simulink model "Trial_Merge_Unsuccessful"  (R2020b)
settings: Solver=VariableStepAuto  StartTime=0.0  StopTime=10.0  RelTol=1e-3
values from neighbouring files (symbols this model uses):
  A_2 = zeros(3)    [MPC_tune.m]
  B_2 = I_inv    [MPC_tune.m]
  C_2 = eye(3)    [MPC_tune.m]
  D_2 = zeros(3)    [MPC_tune.m]
  I_inv = inv(I_mat)    [MPC_tune.m]
undefined symbols (not defined in the file or in its folder): Fb1_l, Fb1_u, Fb2_l, Fb2_u, Fb3_l, Fb3_u, Fb4_l, Fb4_u, Fc1_l, Fc1_u, Fc2_l, Fc2_u, Fc3_l, Fc3_u, fprop, Ft1_l, Ft1_u, Ft2_l, Ft2_u, Ft3_l, Ft3_u, Ft4_l, Ft4_u, theta0
libraries: dspsigops x33, pid_lib x3, fuzblock x3, mpclib x1, dspmathops x1
(part 1 of 2)
settings Model: Creator=Jonathan van Zyl  LastModifiedBy=Jonathan van Zyl

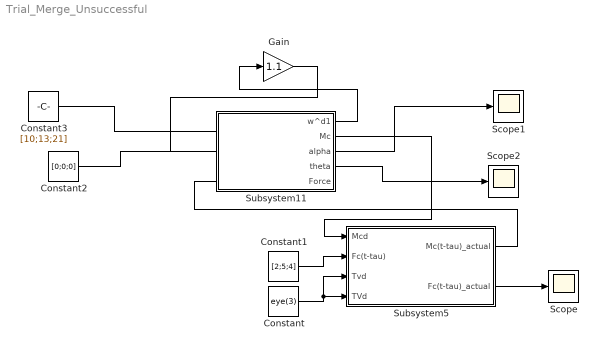
== system Trial_Merge_Unsuccessful ==
  Constant : Constant  Value=eye(3)
  Constant1 : Constant  Value=[2;5;4]
  Constant2 : Constant  Value=[0;0;0]
  Constant3 : Constant  Value=[10;13;21]
  Gain : Gain  Gain=1.1
  Scope : Scope
  Scope1 : Scope
  Scope2 : Scope
  Subsystem11 : Subsystem
  Subsystem5 : Subsystem
  wires:
  Subsystem11/2(Mc) -> Subsystem5/1(Mcd)
  Subsystem5/2(Fc(t-tau)_actual) -> Scope/1
  Constant/1 -> Subsystem5/4(TVd), Subsystem5/3(Tvd)
  Constant1/1 -> Subsystem5/2(Fc(t-tau))
  Subsystem11/1(w^d1) -> Gain/1
  Gain/1 -> ?
  Subsystem5/1(Mc(t-tau)_actual) -> ?
  Constant2/1 -> ?
  Constant3/1 -> ?
  Subsystem11/3(alpha) -> Scope1/1
  Subsystem11/4(theta) -> Scope2/1

== system Trial_Merge_Unsuccessful/Subsystem11 ==
  Add : Sum  Inputs=+++
  Constant : Constant  Value=[0;0;0]
  Constant1 : Constant  Value=[2;3;4]
  Demux : Demux  Outputs=3
  Gain3 : Gain  Gain=180/pi
  M_aero : Constant  Value=[2;3;4]
  Scope : Scope
  Scope1 : Scope
  Scope8 : Scope
  Square : Math  Operator=square  SaturateOnIntegerOverflow=on
  Square Root : Sqrt  SaturateOnIntegerOverflow=on
  Square1 : Math  Operator=square  SaturateOnIntegerOverflow=on
  Square2 : Math  Operator=square  SaturateOnIntegerOverflow=on
  Subsystem : Subsystem
  To Workspace : ToWorkspace  VariableName=angle_deg  SaveFormat=Timeseries  SampleTime=-1
  To Workspace1 : ToWorkspace  VariableName=alpha  SaveFormat=Timeseries  SampleTime=-1
  initial w : Constant  Value=[0;0;0]
  sigma,upsilon,tau : Constant  Value=[2;3;4]
  w^d1 : Outport
  Mc : Outport  Port=2
  alpha : Outport  Port=3
  theta : Outport  Port=4
  Force : Outport  Port=5
  wires:
  Subsystem/4(alpha) -> Demux/1, Scope/1, alpha/1
  Demux/1 -> Square/1
  Demux/2 -> Square1/1
  Demux/3 -> Square2/1
  Square/1 -> Add/1
  Square1/1 -> Add/2
  Square2/1 -> Add/3
  Add/1 -> Square Root/1
  Square Root/1 -> To Workspace1/1, Scope1/1
  sigma,upsilon,tau/1 -> Subsystem/2(sigma,tau,upsilon)
  initial w/1 -> Subsystem/3(initial w)
  M_aero/1 -> Subsystem/1(M_aero)
  Subsystem/3(Mc) -> Mc/1
  Subsystem/2(w_out) -> w^d1/1
  Subsystem/1(theta_out) -> Gain3/1, theta/1
  Gain3/1 -> To Workspace/1, Scope8/1
  Subsystem/5(Force) -> Force/1
  Constant/1 -> Subsystem/4(Fc)
  Constant1/1 -> Subsystem/5(a)

== system Trial_Merge_Unsuccessful/Subsystem5 ==
  Mcd : Inport
  Fc(t-tau) : Inport  Port=2
  Tvd : Inport  Port=3
  TVd : Inport  Port=4
  Gain6 : Gain
  MATLAB Function4 : MATLAB Function  Commented=on  TreatAsAtomicUnit=on
  MATLAB Function5 : MATLAB Function  Commented=on  TreatAsAtomicUnit=on
  Matrix Multiply5 : Product  Multiplication=Matrix(*)
  Scope16 : Scope
  Scope17 : Scope
  Scope18 : Scope
  Subsystem : Subsystem
  Subsystem1 : Subsystem
  Subsystem2 : Subsystem
  Subsystem3 : Subsystem
  Subsystem4 : Subsystem
  Turn off for PID tune : Gain
  Mc(t-tau)_actual : Outport
  Fc(t-tau)_actual : Outport  Port=2
  wires:
  Mcd/1 -> Gain6/1
  Turn off for PID tune/1 -> Matrix Multiply5/2
  Tvd/1 -> Matrix Multiply5/1
  Fc(t-tau)/1 -> Turn off for PID tune/1
  MATLAB Function5/1(F1) -> MATLAB Function4/1(F1)
  MATLAB Function5/3(F3) -> MATLAB Function4/3(F3)
  MATLAB Function5/2(F2) -> MATLAB Function4/2(F2)
  Matrix Multiply5/1 -> Subsystem/1(F_c_d)  "F_c_d"
  Gain6/1 -> Subsystem/2(M_c_d)  "M_c_d"
  Subsystem/1(Fb_wanted) -> Subsystem1/1(In1)
  Subsystem/2(Ft_wanted) -> Subsystem1/2(In2)
  Subsystem/3(Fc_wanted) -> Subsystem1/3(In3)
  Subsystem1/1(Out1) -> Subsystem2/1(In1)
  Subsystem1/2(Out2) -> Subsystem2/2(In2)
  Subsystem1/3(Out3) -> Subsystem2/3(In3)
  Subsystem3/1(Out1) -> Scope17/1, Subsystem4/2(In2)
  Subsystem2/1(F_c_max) -> Subsystem3/1(In1)
  Subsystem2/2(F_t_max) -> Subsystem3/2(In2)
  Subsystem2/3(Out3) -> Subsystem3/3(In3)
  Subsystem2/4(Out4) -> Subsystem3/4(Ft3)
  Subsystem2/5(Out5) -> Subsystem3/5(Ft4)
  Subsystem2/6(Out6) -> Subsystem3/6(Fb1)
  Subsystem2/7(Out7) -> Subsystem3/7(In7)
  Subsystem2/8(Out8) -> Subsystem3/8(Fb3)
  Subsystem2/9(Out9) -> Subsystem3/9(In9)
  Subsystem3/2(Mc(t-tau)_actual) -> Mc(t-tau)_actual/1
  Subsystem4/1(Fc(t-tau)_actual) -> Scope16/1, Fc(t-tau)_actual/1
  TVd/1 -> Subsystem4/1(TVd)
  Subsystem4/2(Fc(t-tau)_actual1) -> Scope18/1

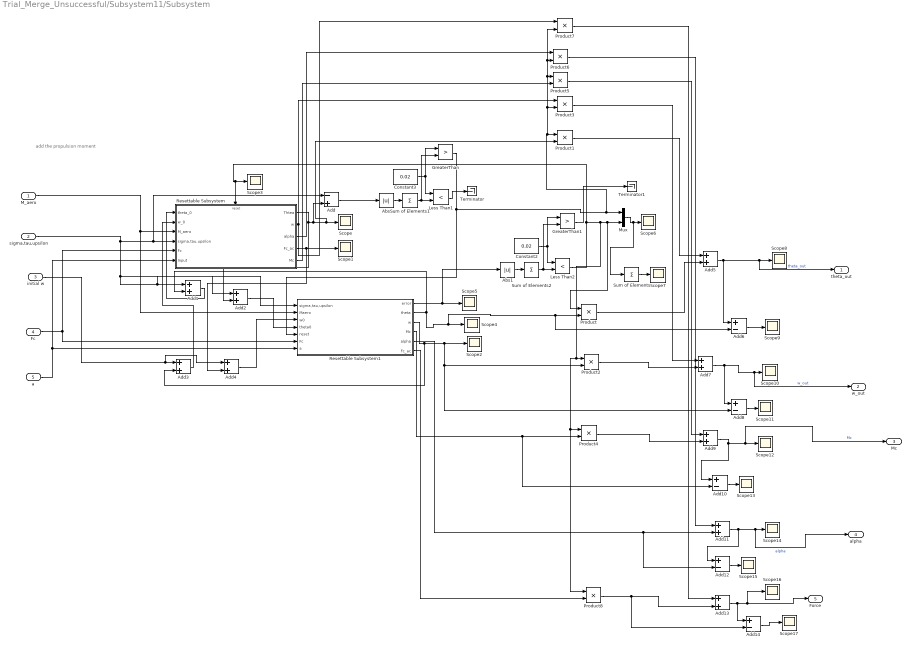
== system Trial_Merge_Unsuccessful/Subsystem11/Subsystem ==
  note: add the propulsion moment
  M_aero : Inport
  sigma,tau,upsilon : Inport  Port=2
  initial w : Inport  Port=3
  Fc : Inport  Port=4
  a : Inport  Port=5
  Abs : Abs
  Abs1 : Abs
  Add : Sum  Inputs=-+
  Add{1..5,7,9,11,13} (9 alike) : Sum
  Add{6,8,10,12,14} (5 alike) : Sum  Inputs=+-
  Constant2 : Constant  Value=0.02
  Constant3 : Constant  Value=0.02
  GreaterThan : RelationalOperator  Operator=>  OutDataTypeStr=boolean  RndMeth=Simplest
  GreaterThan1 : RelationalOperator  Operator=>  OutDataTypeStr=boolean  RndMeth=Simplest
  Less Than1 : RelationalOperator  Operator=<  OutDataTypeStr=boolean  RndMeth=Simplest
  Less Than2 : RelationalOperator  Operator=<  OutDataTypeStr=boolean  RndMeth=Simplest
  Mux : Mux  Inputs=2
  Product{,1..8} (9 alike) : Product
  Resettable Subsystem : Subsystem  TreatAsAtomicUnit=on
  Resettable Subsystem1 : Subsystem  TreatAsAtomicUnit=on
  Scope{,1..17} (18 alike) : Scope
  Sum of Elements : Sum  Inputs=+
  Sum of Elements1 : Sum  Inputs=+
  Sum of Elements2 : Sum  Inputs=+
  Terminator : Terminator
  Terminator1 : Terminator
  theta_out : Outport
  w_out : Outport  Port=2
  Mc : Outport  Port=3
  alpha : Outport  Port=4
  Force : Outport  Port=5
  wires:
  Add8/1 -> Scope11/1
  GreaterThan/1 -> Product7/2, Product6/2, Product5/1, Product3/2, Product1/1, Mux/1, Resettable Subsystem1/5(reset)
  Add6/1 -> Scope9/1
  Abs1/1 -> Sum of Elements2/1
  Product1/1 -> Add5/1
  Resettable Subsystem/2(w) -> Scope1/1, Add4/2, Product3/1
  Resettable Subsystem1/4(Mc) -> Add10/2, Product4/2
  Resettable Subsystem1/2(theta) -> Add1/2, Add6/2, Product/2, Scope4/1
  Resettable Subsystem1/5(alpha) -> Add12/2, Add11/2
  Resettable Subsystem/1(Thtea) -> Add2/2, Add/2, Product1/2, Scope/1
  Less Than2/1 -> Product2/1, Product8/1, Product4/1, Product/1, Mux/2, Scope3/1, Resettable Subsystem/Reset
  M_aero/1 -> Resettable Subsystem1/2(Maero), Resettable Subsystem/3(M_aero)
  Resettable Subsystem1/1(error) -> Abs1/1, Scope5/1
  Add11/1 -> Add12/1, alpha/1, Scope14/1  "alpha"
  Product2/1 -> Add7/2
  Constant2/1 -> GreaterThan1/1, Less Than2/1
  Resettable Subsystem1/3(w) -> Add3/2, Scope2/1, Add8/2, Product2/2
  Product3/1 -> Add7/1
  Add12/1 -> Scope15/1
  Abs/1 -> Sum of Elements1/1
  Add5/1 -> Add6/1, theta_out/1, Scope8/1  "theta_out"
  Add2/1 -> Resettable Subsystem1/4(theta0)
  Constant3/1 -> GreaterThan/1, Less Than1/1
  Sum of Elements1/1 -> Less Than1/2, GreaterThan/2
  Add3/1 -> Resettable Subsystem/2(w_0)
  sigma,tau,upsilon/1 -> Add2/1, Add1/1, Resettable Subsystem1/1(sigma,tau,upsilon), Add/1, Resettable Subsystem/4(sigma,tau,upsilon)
  Product5/1 -> Add9/1
  Resettable Subsystem/5(Mc) -> Product5/2
  Add7/1 -> Add8/1, w_out/1, Scope10/1  "w_out"
  Product6/1 -> Add11/1
  Add9/1 -> Add10/1, Mc/1, Scope12/1  "Mc"
  Add/1 -> Abs/1
  Add1/1 -> Resettable Subsystem/1(theta_0)
  Sum of Elements/1 -> Scope7/1
  Sum of Elements2/1 -> Less Than2/2, GreaterThan1/2
  Mux/1 -> Sum of Elements/1, Scope6/1
  Resettable Subsystem/3(alpha) -> Product6/1
  Add4/1 -> Resettable Subsystem1/3(w0)
  initial w/1 -> Add4/1, Add3/1
  Product/1 -> Add5/2
  Add10/1 -> Scope13/1
  Product4/1 -> Add9/2
  GreaterThan1/1 -> Terminator1/1
  Less Than1/1 -> Terminator/1
  Resettable Subsystem/4(Fc_ac) -> Product7/1
  Fc/1 -> Resettable Subsystem/5(Fc), Resettable Subsystem1/6(Fc)
  a/1 -> Resettable Subsystem1/7(a), Resettable Subsystem/6(Input)
  Resettable Subsystem1/6(Fc_ac) -> Product8/2
  Product8/1 -> Add14/2, Add13/2
  Product7/1 -> Add13/1
  Add13/1 -> Add14/1, Force/1, Scope16/1
  Add14/1 -> Scope17/1

== system Trial_Merge_Unsuccessful/Subsystem5/Subsystem ==
  F_c_d : Inport
  M_c_d : Inport  Port=2
  Demux8 : Demux  Outputs=3
  Demux9 : Demux  Outputs=3
  MATLAB Function : MATLAB Function  TreatAsAtomicUnit=on
  MATLAB Function6 : MATLAB Function  TreatAsAtomicUnit=on
  Mux23 : Mux
  Mux24 : Mux
  Mux9 : Mux  Inputs=3
  Terminator12 : Terminator
  To Workspace6 : ToWorkspace  VariableName=Fc_wanted  SaveFormat=Timeseries  SampleTime=-1
  To Workspace7 : ToWorkspace  VariableName=Ft_wanted  SaveFormat=Timeseries  SampleTime=-1
  To Workspace8 : ToWorkspace  VariableName=Fb_wanted  SaveFormat=Timeseries  SampleTime=-1
  Fb_wanted : Outport
  Ft_wanted : Outport  Port=2
  Fc_wanted : Outport  Port=3
  wires:
  Demux9/3 -> MATLAB Function6/3(M_z)
  Demux8/2 -> MATLAB Function6/1(F_y)
  Mux9/1 -> Fc_wanted/1, To Workspace6/1  "Fc_wanted"
  MATLAB Function/2(Ft2) -> Mux23/2  "Fb_wanted"
  Demux9/1 -> MATLAB Function6/2(M_x)
  MATLAB Function/3(Ft3) -> Mux23/3
  Demux9/2 -> MATLAB Function/1(My)
  MATLAB Function/8(Fb4) -> Mux24/4
  MATLAB Function6/1(F_c1) -> Mux9/1
  MATLAB Function/1(Ft1) -> Mux23/1  "Ft_wanted"
  Demux8/1 -> Terminator12/1
  Mux23/1 -> Ft_wanted/1, To Workspace7/1  "Ft_wanted"
  Mux24/1 -> Fb_wanted/1, To Workspace8/1  "Fb_wanted"
  MATLAB Function6/3(F_c3) -> Mux9/3
  MATLAB Function/5(Fb1) -> Mux24/1
  MATLAB Function/6(Fb2) -> Mux24/2
  MATLAB Function/7(Fb3) -> Mux24/3
  MATLAB Function/4(Ft4) -> Mux23/4
  Demux8/3 -> MATLAB Function/2(Fz)
  MATLAB Function6/2(F_c2) -> Mux9/2
  F_c_d/1 -> Demux8/1
  M_c_d/1 -> Demux9/1

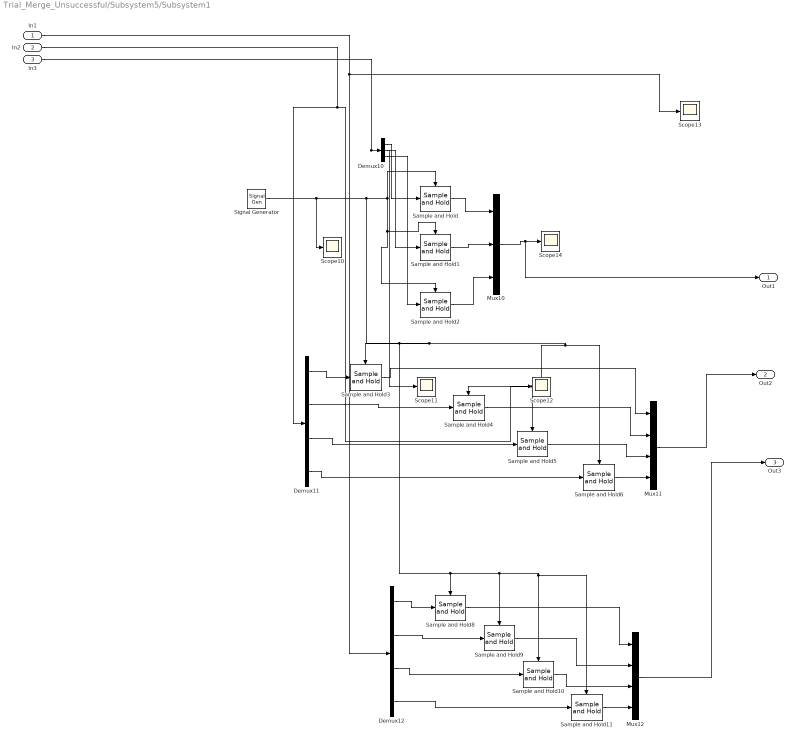
== system Trial_Merge_Unsuccessful/Subsystem5/Subsystem1 ==
  In1 : Inport
  In2 : Inport  Port=2
  In3 : Inport  Port=3
  Demux10 : Demux  Outputs=3
  Demux11 : Demux
  Demux12 : Demux
  Mux10 : Mux  Inputs=3
  Mux11 : Mux
  Mux12 : Mux
  Sample and Hold{,1..6,8..11} (11 alike) : dspsigops/Sample and Hold  trig=Rising edge  initCond=0  latchinput=off
  Scope{10..14} (5 alike) : Scope
  Signal Generator : SignalGenerator  WaveForm=square  Frequency=fprop  Units=rad/sec
  Out1 : Outport
  Out2 : Outport  Port=2
  Out3 : Outport  Port=3
  wires:
  Demux12/1 -> Sample and Hold8/1
  Demux11/1 -> Sample and Hold3/1
  Signal Generator/1 -> Scope10/1, Sample and Hold11/Trigger, Sample and Hold10/Trigger, Sample and Hold9/Trigger, Sample and Hold8/Trigger, Sample and Hold4/Trigger, Sample and Hold5/Trigger, Sample and Hold6/Trigger, Sample and Hold3/Trigger, Sample and Hold/Trigger, Sample and Hold2/Trigger, Sample and Hold1/Trigger
  In2/1 -> Scope12/1, Demux11/1
  In3/1 -> Scope11/1, Demux10/1
  Demux10/3 -> Sample and Hold2/1
  Sample and Hold10/1 -> Mux12/3
  Sample and Hold/1 -> Mux10/1
  Demux12/4 -> Sample and Hold11/1
  Sample and Hold6/1 -> Mux11/4
  Demux10/1 -> Sample and Hold/1
  Mux10/1 -> Out1/1, Scope14/1
  Demux12/3 -> Sample and Hold10/1
  Sample and Hold8/1 -> Mux12/1
  Sample and Hold3/1 -> Mux11/1
  Sample and Hold5/1 -> Mux11/3
  Sample and Hold1/1 -> Mux10/2
  Sample and Hold11/1 -> Mux12/4
  In1/1 -> Scope13/1, Demux12/1
  Demux10/2 -> Sample and Hold1/1
  Demux11/2 -> Sample and Hold4/1
  Sample and Hold2/1 -> Mux10/3
  Sample and Hold4/1 -> Mux11/2
  Sample and Hold9/1 -> Mux12/2
  Demux11/3 -> Sample and Hold5/1
  Mux12/1 -> Out3/1
  Demux12/2 -> Sample and Hold9/1
  Demux11/4 -> Sample and Hold6/1
  Mux11/1 -> Out2/1

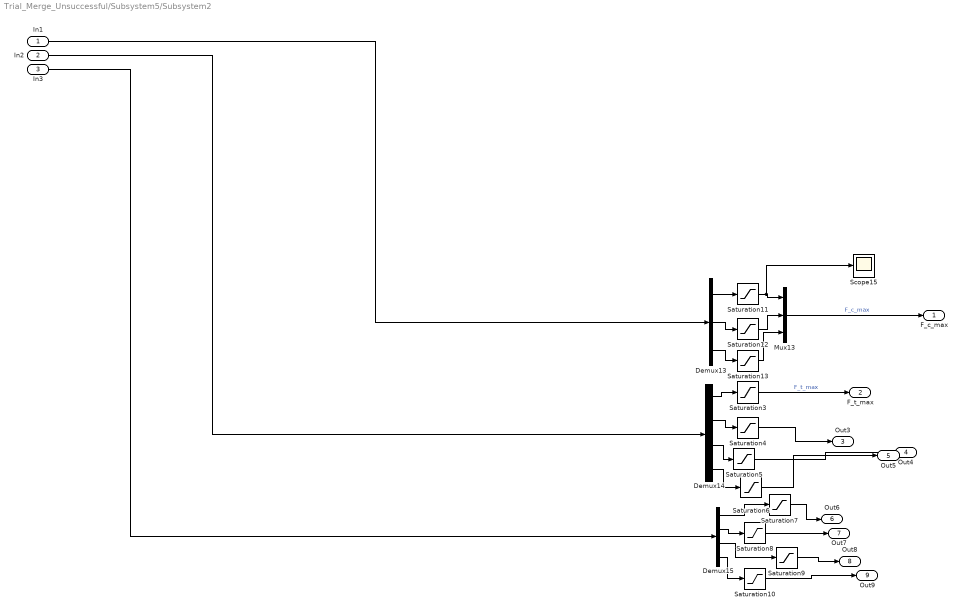
== system Trial_Merge_Unsuccessful/Subsystem5/Subsystem2 ==
  In1 : Inport
  In2 : Inport  Port=2
  In3 : Inport  Port=3
  Demux13 : Demux  Outputs=3
  Demux14 : Demux
  Demux15 : Demux
  Mux13 : Mux  Inputs=3
  Saturation10 : Saturate  UpperLimit=Fb4_u  LowerLimit=Fb4_l
  Saturation11 : Saturate  UpperLimit=Fc1_u  LowerLimit=Fc1_l
  Saturation12 : Saturate  UpperLimit=Fc2_u  LowerLimit=Fc2_l
  Saturation13 : Saturate  UpperLimit=Fc3_u  LowerLimit=Fc3_l
  Saturation3 : Saturate  UpperLimit=Ft1_u  LowerLimit=Ft1_l
  Saturation4 : Saturate  UpperLimit=Ft2_u  LowerLimit=Ft2_l
  Saturation5 : Saturate  UpperLimit=Ft3_u  LowerLimit=Ft3_l
  Saturation6 : Saturate  UpperLimit=Ft4_u  LowerLimit=Ft4_l
  Saturation7 : Saturate  UpperLimit=Fb1_u  LowerLimit=Fb1_l
  Saturation8 : Saturate  UpperLimit=Fb2_u  LowerLimit=Fb2_l
  Saturation9 : Saturate  UpperLimit=Fb3_u  LowerLimit=Fb3_l
  Scope15 : Scope
  F_c_max : Outport
  F_t_max : Outport  Port=2
  Out3 : Outport  Port=3
  Out4 : Outport  Port=4
  Out5 : Outport  Port=5
  Out6 : Outport  Port=6
  Out7 : Outport  Port=7
  Out8 : Outport  Port=8
  Out9 : Outport  Port=9
  wires:
  Saturation11/1 -> Scope15/1, Mux13/1
  Demux13/2 -> Saturation12/1
  Saturation10/1 -> Out9/1
  Demux13/3 -> Saturation13/1
  Demux14/1 -> Saturation3/1
  Demux14/4 -> Saturation6/1
  In3/1 -> Demux15/1
  Demux14/3 -> Saturation5/1
  Demux13/1 -> Saturation11/1
  Saturation13/1 -> Mux13/3
  In1/1 -> Demux13/1
  Demux15/1 -> Saturation7/1
  Demux15/2 -> Saturation8/1
  Demux15/3 -> Saturation9/1
  Saturation12/1 -> Mux13/2
  Demux15/4 -> Saturation10/1
  Demux14/2 -> Saturation4/1
  Saturation9/1 -> Out8/1
  Saturation5/1 -> Out4/1
  In2/1 -> Demux14/1
  Saturation4/1 -> Out3/1
  Saturation7/1 -> Out6/1
  Mux13/1 -> F_c_max/1  "F_c_max"
  Saturation6/1 -> Out5/1
  Saturation3/1 -> F_t_max/1  "F_t_max"
  Saturation8/1 -> Out7/1

== system Trial_Merge_Unsuccessful/Subsystem5/Subsystem3 ==
  In1 : Inport
  In2 : Inport  Port=2
  In3 : Inport  Port=3
  Ft3 : Inport  Port=4
  Ft4 : Inport  Port=5
  Fb1 : Inport  Port=6
  In7 : Inport  Port=7
  Fb3 : Inport  Port=8
  In9 : Inport  Port=9
  Constant23 : Constant  Value=0
  Demux16 : Demux  Outputs=3
  MATLAB Function7 : MATLAB Function  TreatAsAtomicUnit=on
  MATLAB Function8 : MATLAB Function  TreatAsAtomicUnit=on
  MATLAB Function9 : MATLAB Function  TreatAsAtomicUnit=on
  Mux : Mux
  Mux1 : Mux
  Mux16 : Mux  Inputs=3
  Mux17 : Mux  Inputs=3
  To Workspace : ToWorkspace  VariableName=Fc  SaveFormat=Timeseries  SampleTime=-1
  To Workspace1 : ToWorkspace  VariableName=Ft  SaveFormat=Timeseries  SampleTime=-1
  To Workspace2 : ToWorkspace  VariableName=Fb  SaveFormat=Timeseries  SampleTime=-1
  Out1 : Outport
  Mc(t-tau)_actual : Outport  Port=2
  wires:
  Demux16/2 -> MATLAB Function8/2(F_c2)
  In9/1 -> Mux1/4, MATLAB Function9/8(Fb4)
  In3/1 -> Mux/2, MATLAB Function9/2(Ft2)
  MATLAB Function7/1(F_z) -> Mux16/3  "Fz_actual"
  In1/1 -> Demux16/1, To Workspace/1
  Fb3/1 -> Mux1/3, MATLAB Function9/7(Fb3)
  MATLAB Function9/1(F1) -> MATLAB Function7/1(F1)
  Ft3/1 -> Mux/3, MATLAB Function9/3(Ft3)
  MATLAB Function8/1(F_y) -> Mux16/2  "Fy_actual"
  Fb1/1 -> Mux1/1, MATLAB Function9/5(Fb1)
  MATLAB Function8/3(M_z) -> Mux17/3  "M_z_acc"
  MATLAB Function7/2(M_y) -> Mux17/2  "M_y_acc"
  Mux17/1 -> Mc(t-tau)_actual/1  "Mc(t-tau)_actual"
  Ft4/1 -> Mux/4, MATLAB Function9/4(Ft4)
  MATLAB Function8/2(M_x) -> Mux17/1  "M_x_acc"
  In7/1 -> Mux1/2, MATLAB Function9/6(Fb2)
  MATLAB Function9/3(F3) -> MATLAB Function7/3(F3)
  Demux16/1 -> MATLAB Function8/1(F_c1)
  Constant23/1 -> Mux16/1  "Fx_actual"
  In2/1 -> Mux/1, MATLAB Function9/1(Ft1)
  MATLAB Function9/2(F2) -> MATLAB Function7/2(F2)
  Mux1/1 -> To Workspace2/1
  Demux16/3 -> MATLAB Function8/3(F_c3)
  Mux/1 -> To Workspace1/1
  Mux16/1 -> Out1/1

== system Trial_Merge_Unsuccessful/Subsystem5/Subsystem4 ==
  TVd : Inport
  In2 : Inport  Port=2
  Constant24 : Constant  Value=[0;1;1]
  Matrix Multiply3 : Product  Multiplication=Matrix(*)
  Product5 : Product
  Fc(t-tau)_actual : Outport
  Fc(t-tau)_actual1 : Outport  Port=2
  wires:
  Matrix Multiply3/1 -> Fc(t-tau)_actual1/1, Product5/2  "Fc(t-tau)_actual"
  Constant24/1 -> Product5/1
  TVd/1 -> Matrix Multiply3/1
  Product5/1 -> Fc(t-tau)_actual/1  "Fc(t-tau)_actual"
  In2/1 -> Matrix Multiply3/2

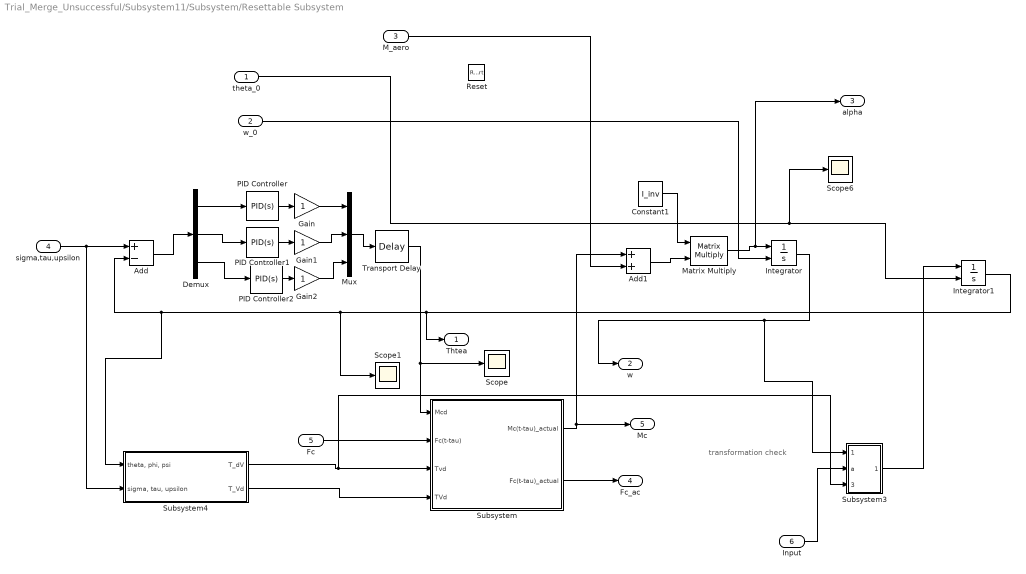
== system Trial_Merge_Unsuccessful/Subsystem11/Subsystem/Resettable Subsystem ==
  note: transformation check
  theta_0 : Inport
  w_0 : Inport  Port=2
  M_aero : Inport  Port=3
  sigma,tau,upsilon : Inport  Port=4
  Fc : Inport  Port=5
  Input : Inport  Port=6
  Reset : ResetPort  DisableCoverage=on  ResetTriggerType=either
  Add : Sum  Inputs=+-
  Add1 : Sum
  Constant1 : Constant  Value=I_inv
  Demux : Demux  Outputs=3
  Gain : Gain
  Gain1 : Gain
  Gain2 : Gain
  Integrator : Integrator  InitialConditionSource=external  InitialCondition=[0.15;-0.2;0.01]
  Integrator1 : Integrator  InitialConditionSource=external  InitialCondition=[0.01;-0.01;0.005]
  Matrix Multiply : Product  Multiplication=Matrix(*)
  Mux : Mux  Inputs=3
  PID Controller : pid_lib/PID Controller  Controller=PID  Form=Parallel  TimeDomain=Continuous-time  UseExternalTs=off  SampleTime=-1  IntegratorMethod=Forward Euler  FilterMethod=Forward Euler  ControllerParametersSource=internal  P=76.4274415550338  I=3.57793373088927  D=400.875615235633  UseFilter=on  N=5.45397025421619  TunerSelectOption=Transfer Function Based (PID Tuner App)  InitialConditionSource=internal  InitialConditionForIntegrator=0  InitialConditionForFilter=0  DifferentiatorICPrevScaledInput=0  ExternalReset=none  TrackingMode=off  Kt=1  LimitOutput=off  SatLimitsSource=internal  UpperSaturationLimit=inf  LowerSaturationLimit=-inf  LinearizeAsGain=on  AntiWindupMode=none  Kb=1  POutMin=[]  POutMax=[]  IOutMin=[]  IOutMax=[]  DOutMin=[]  DOutMax=[]  NOutMin=[]  NOutMax=[]  SumOutMin=[]  SumOutMax=[]  SaturationOutMin=[]  SaturationOutMax=[]  PParamMin=[]  PParamMax=[]  IParamMin=[]  IParamMax=[]  DParamMin=[]  DParamMax=[]  NParamMin=[]  NParamMax=[]  KbParamMin=[]  KbParamMax=[]  KtParamMin=[]  KtParamMax=[]  KbOutMin=[]  KbOutMax=[]  KtOutMin=[]  KtOutMax=[]  IntegratorOutMin=[]  IntegratorOutMax=[]  FilterOutMin=[]  FilterOutMax=[]  SumI1OutMin=[]  SumI1OutMax=[]  SumI2OutMin=[]  SumI2OutMax=[]  SumI3OutMin=[]  SumI3OutMax=[]  SumI4OutMin=[]  SumI4OutMax=[]  SumDOutMin=[]  SumDOutMax=[]  DifferentiatorOutMin=[]  DifferentiatorOutMax=[]  FilterDiffOutCoefMin=[]  FilterDiffOutCoefMax=[]  ReciprocalOutMin=[]  ReciprocalOutMax=[]  SumDenOutMin=[]  SumDenOutMax=[]  SumNumOutMin=[]  SumNumOutMax=[]  DivideOutMin=[]  DivideOutMax=[]  UdiffTsProdOutMin=[]  UdiffTsProdOutMax=[]  NTsProdOutMin=[]  NTsProdOutMax=[]  UintegralTsProdOutMin=[]  UintegralTsProdOutMax=[]  UngainTsProdOutMin=[]  UngainTsProdOutMax=[]  IntegratorContinuousStateAttributes=''  IntegratorStateMustResolveToSignalObject=off  IntegratorRTWStateStorageClass=Auto  FilterContinuousStateAttributes=''  FilterStateMustResolveToSignalObject=off  FilterRTWStateStorageClass=Auto  ParallelPVariant=InternalParameters  IdealPVariant=Disabled  IVariant=InternalParameters  DVariant=InternalParameters  IntegratorVariant=Continuous  SatVariant=Disabled  AWVariant=Passthrough  PCopyVariant=Disabled  TRVariant=Disabled  FdbkBlocksVariant=Forward  IdealPFdbkVariant=Disabled  SatFdbkVariant=Disabled  DerivativeFilterVariant=ContFilter  NVariant=InternalParameters  NCopyVariant=Disabled  FilterICVariant=InternalICsFilter  IntegratorICVariant=InternalICs  ExternalResetVariant=Disabled  TRSumVariant=Passthrough  SumFdbkVariant=Disabled  SumVariant=Sum_PID  TsampFilterVariant=InternalTs  TsampNgainVariant=Passthrough  TsampIntegralVariant=Passthrough  ExternalSaturationOutDataTypeStr=Inherit: Same as second input
  PID Controller1 : pid_lib/PID Controller  Controller=PID  Form=Parallel  TimeDomain=Continuous-time  UseExternalTs=off  SampleTime=-1  IntegratorMethod=Forward Euler  FilterMethod=Forward Euler  ControllerParametersSource=internal  P=-202.527799620363  I=-9.48129403471772  D=-1062.29457146841  UseFilter=on  N=5.45397025421619  TunerSelectOption=Transfer Function Based (PID Tuner App)  InitialConditionSource=internal  InitialConditionForIntegrator=0  InitialConditionForFilter=0  DifferentiatorICPrevScaledInput=0  ExternalReset=none  TrackingMode=off  Kt=1  LimitOutput=off  SatLimitsSource=internal  UpperSaturationLimit=inf  LowerSaturationLimit=-inf  LinearizeAsGain=on  AntiWindupMode=none  Kb=1  POutMin=[]  POutMax=[]  IOutMin=[]  IOutMax=[]  DOutMin=[]  DOutMax=[]  NOutMin=[]  NOutMax=[]  SumOutMin=[]  SumOutMax=[]  SaturationOutMin=[]  SaturationOutMax=[]  PParamMin=[]  PParamMax=[]  IParamMin=[]  IParamMax=[]  DParamMin=[]  DParamMax=[]  NParamMin=[]  NParamMax=[]  KbParamMin=[]  KbParamMax=[]  KtParamMin=[]  KtParamMax=[]  KbOutMin=[]  KbOutMax=[]  KtOutMin=[]  KtOutMax=[]  IntegratorOutMin=[]  IntegratorOutMax=[]  FilterOutMin=[]  FilterOutMax=[]  SumI1OutMin=[]  SumI1OutMax=[]  SumI2OutMin=[]  SumI2OutMax=[]  SumI3OutMin=[]  SumI3OutMax=[]  SumI4OutMin=[]  SumI4OutMax=[]  SumDOutMin=[]  SumDOutMax=[]  DifferentiatorOutMin=[]  DifferentiatorOutMax=[]  FilterDiffOutCoefMin=[]  FilterDiffOutCoefMax=[]  ReciprocalOutMin=[]  ReciprocalOutMax=[]  SumDenOutMin=[]  SumDenOutMax=[]  SumNumOutMin=[]  SumNumOutMax=[]  DivideOutMin=[]  DivideOutMax=[]  UdiffTsProdOutMin=[]  UdiffTsProdOutMax=[]  NTsProdOutMin=[]  NTsProdOutMax=[]  UintegralTsProdOutMin=[]  UintegralTsProdOutMax=[]  UngainTsProdOutMin=[]  UngainTsProdOutMax=[]  IntegratorContinuousStateAttributes=''  IntegratorStateMustResolveToSignalObject=off  IntegratorRTWStateStorageClass=Auto  FilterContinuousStateAttributes=''  FilterStateMustResolveToSignalObject=off  FilterRTWStateStorageClass=Auto  ParallelPVariant=InternalParameters  IdealPVariant=Disabled  IVariant=InternalParameters  DVariant=InternalParameters  IntegratorVariant=Continuous  SatVariant=Disabled  AWVariant=Passthrough  PCopyVariant=Disabled  TRVariant=Disabled  FdbkBlocksVariant=Forward  IdealPFdbkVariant=Disabled  SatFdbkVariant=Disabled  DerivativeFilterVariant=ContFilter  NVariant=InternalParameters  NCopyVariant=Disabled  FilterICVariant=InternalICsFilter  IntegratorICVariant=InternalICs  ExternalResetVariant=Disabled  TRSumVariant=Passthrough  SumFdbkVariant=Disabled  SumVariant=Sum_PID  TsampFilterVariant=InternalTs  TsampNgainVariant=Passthrough  TsampIntegralVariant=Passthrough  ExternalSaturationOutDataTypeStr=Inherit: Same as second input
  PID Controller2 : pid_lib/PID Controller  Controller=PID  Form=Parallel  TimeDomain=Continuous-time  UseExternalTs=off  SampleTime=-1  IntegratorMethod=Forward Euler  FilterMethod=Forward Euler  ControllerParametersSource=internal  P=-232.294042315359  I=-10.8747940867059  D=-1218.42384402842  UseFilter=on  N=5.45397025421619  TunerSelectOption=Transfer Function Based (PID Tuner App)  InitialConditionSource=internal  InitialConditionForIntegrator=0  InitialConditionForFilter=0  DifferentiatorICPrevScaledInput=0  ExternalReset=none  TrackingMode=off  Kt=1  LimitOutput=off  SatLimitsSource=internal  UpperSaturationLimit=inf  LowerSaturationLimit=-inf  LinearizeAsGain=on  AntiWindupMode=none  Kb=1  POutMin=[]  POutMax=[]  IOutMin=[]  IOutMax=[]  DOutMin=[]  DOutMax=[]  NOutMin=[]  NOutMax=[]  SumOutMin=[]  SumOutMax=[]  SaturationOutMin=[]  SaturationOutMax=[]  PParamMin=[]  PParamMax=[]  IParamMin=[]  IParamMax=[]  DParamMin=[]  DParamMax=[]  NParamMin=[]  NParamMax=[]  KbParamMin=[]  KbParamMax=[]  KtParamMin=[]  KtParamMax=[]  KbOutMin=[]  KbOutMax=[]  KtOutMin=[]  KtOutMax=[]  IntegratorOutMin=[]  IntegratorOutMax=[]  FilterOutMin=[]  FilterOutMax=[]  SumI1OutMin=[]  SumI1OutMax=[]  SumI2OutMin=[]  SumI2OutMax=[]  SumI3OutMin=[]  SumI3OutMax=[]  SumI4OutMin=[]  SumI4OutMax=[]  SumDOutMin=[]  SumDOutMax=[]  DifferentiatorOutMin=[]  DifferentiatorOutMax=[]  FilterDiffOutCoefMin=[]  FilterDiffOutCoefMax=[]  ReciprocalOutMin=[]  ReciprocalOutMax=[]  SumDenOutMin=[]  SumDenOutMax=[]  SumNumOutMin=[]  SumNumOutMax=[]  DivideOutMin=[]  DivideOutMax=[]  UdiffTsProdOutMin=[]  UdiffTsProdOutMax=[]  NTsProdOutMin=[]  NTsProdOutMax=[]  UintegralTsProdOutMin=[]  UintegralTsProdOutMax=[]  UngainTsProdOutMin=[]  UngainTsProdOutMax=[]  IntegratorContinuousStateAttributes=''  IntegratorStateMustResolveToSignalObject=off  IntegratorRTWStateStorageClass=Auto  FilterContinuousStateAttributes=''  FilterStateMustResolveToSignalObject=off  FilterRTWStateStorageClass=Auto  ParallelPVariant=InternalParameters  IdealPVariant=Disabled  IVariant=InternalParameters  DVariant=InternalParameters  IntegratorVariant=Continuous  SatVariant=Disabled  AWVariant=Passthrough  PCopyVariant=Disabled  TRVariant=Disabled  FdbkBlocksVariant=Forward  IdealPFdbkVariant=Disabled  SatFdbkVariant=Disabled  DerivativeFilterVariant=ContFilter  NVariant=InternalParameters  NCopyVariant=Disabled  FilterICVariant=InternalICsFilter  IntegratorICVariant=InternalICs  ExternalResetVariant=Disabled  TRSumVariant=Passthrough  SumFdbkVariant=Disabled  SumVariant=Sum_PID  TsampFilterVariant=InternalTs  TsampNgainVariant=Passthrough  TsampIntegralVariant=Passthrough  ExternalSaturationOutDataTypeStr=Inherit: Same as second input
  Scope : Scope
  Scope1 : Scope
  Scope6 : Scope
  Subsystem : Subsystem
  Subsystem3 : Subsystem
  Subsystem4 : Subsystem
  Transport Delay : TransportDelay  DelayTime=0.1
  Thtea : Outport
  w : Outport  Port=2
  alpha : Outport  Port=3
  Fc_ac : Outport  Port=4
  Mc : Outport  Port=5
  wires:
  Transport Delay/1 -> Subsystem/1(Mcd), Scope/1
  Constant1/1 -> Matrix Multiply/1
  PID Controller2/1 -> Gain2/1
  PID Controller/1 -> Gain/1
  Matrix Multiply/1 -> alpha/1, Integrator/1
  Demux/3 -> PID Controller2/1
  Mux/1 -> Transport Delay/1
  sigma,tau,upsilon/1 -> Subsystem4/2("sigma, tau, upsilon"), Add/1
  Gain/1 -> Mux/1
  w_0/1 -> Integrator/2
  Gain2/1 -> Mux/3
  Add/1 -> Demux/1
  Add1/1 -> Matrix Multiply/2
  PID Controller1/1 -> Gain1/1
  Integrator/1 -> Subsystem3/1(w^d), w/1
  theta_0/1 -> Integrator1/2, Scope6/1
  Demux/2 -> PID Controller1/1
  Gain1/1 -> Mux/2
  M_aero/1 -> Add1/2
  Demux/1 -> PID Controller/1
  Integrator1/1 -> Thtea/1, Scope1/1, Subsystem4/1("theta, phi, psi"), Add/2
  Subsystem/1(Mc(t-tau)_actual) -> Add1/1, Mc/1
  Subsystem3/1(w^d1) -> Integrator1/1
  Subsystem/2(Fc(t-tau)_actual) -> Fc_ac/1
  Fc/1 -> Subsystem/2(Fc(t-tau))
  Subsystem4/1(T_dV) -> Subsystem3/3(T_dV), Subsystem/3(Tvd)
  Subsystem4/2(T_Vd) -> Subsystem/4(TVd)
  Input/1 -> Subsystem3/2(a)

== system Trial_Merge_Unsuccessful/Subsystem11/Subsystem/Resettable Subsystem1 ==
  sigma,tau,upsilon : Inport
  Maero : Inport  Port=2
  w0 : Inport  Port=3
  theta0 : Inport  Port=4
  reset : Inport  Port=5
  Fc : Inport  Port=6
  a : Inport  Port=7
  Add : Sum  Inputs=-+
  Subsystem : Subsystem
  Subsystem1 : Subsystem
  Subsystem3 : Subsystem
  Subsystem4 : Subsystem
  error : Outport
  theta : Outport  Port=2
  w : Outport  Port=3
  Mc : Outport  Port=4
  alpha : Outport  Port=5
  Fc_ac : Outport  Port=6
  wires:
  theta0/1 -> Subsystem/4(tehat0)
  Subsystem/2(w) -> Subsystem3/1(w^d), w/1
  Add/1 -> error/1
  Maero/1 -> Subsystem/1(M_aero)
  sigma,tau,upsilon/1 -> Subsystem4/2("sigma, tau, upsilon"), Add/2, Subsystem/2(sigma,tau,upsilon)  "sigma, tau, upsilon"
  Subsystem/1(theta) -> Add/1, Subsystem4/1("theta, phi, psi"), theta/1
  w0/1 -> Subsystem/3(w0)
  reset/1 -> Subsystem/5(reset)
  Subsystem/3(Mc) -> Subsystem1/1(Mcd), Mc/1
  Subsystem/4(alpha) -> alpha/1
  Subsystem4/1(T_dV) -> Subsystem3/3(T_dV), Subsystem1/3(Tvd)
  Subsystem1/2(Fc(t-tau)_actual) -> Fc_ac/1
  Subsystem4/2(T_Vd) -> Subsystem1/4(TVd)
  a/1 -> Subsystem3/2(a)
  Subsystem1/1(Mc(t-tau)_actual) -> Subsystem/6(Mprop)
  Fc/1 -> Subsystem1/2(Fc(t-tau))
  Subsystem3/1(w^d1) -> Subsystem/7(wsensed)

== system Trial_Merge_Unsuccessful/Subsystem11/Subsystem/Resettable Subsystem/Subsystem ==
  Mcd : Inport
  Fc(t-tau) : Inport  Port=2
  Tvd : Inport  Port=3
  TVd : Inport  Port=4
  Gain6 : Gain
  MATLAB Function4 : MATLAB Function  Commented=on  TreatAsAtomicUnit=on
  MATLAB Function5 : MATLAB Function  Commented=on  TreatAsAtomicUnit=on
  Matrix Multiply5 : Product  Multiplication=Matrix(*)
  Scope16 : Scope
  Scope17 : Scope
  Scope18 : Scope
  Subsystem : Subsystem
  Subsystem1 : Subsystem
  Subsystem2 : Subsystem
  Subsystem3 : Subsystem
  Subsystem4 : Subsystem
  Turn off for PID tune : Gain
  Mc(t-tau)_actual : Outport
  Fc(t-tau)_actual : Outport  Port=2
  wires:
  Gain6/1 -> Subsystem/2(M_c_d)  "M_c_d"
  Tvd/1 -> Matrix Multiply5/1
  Subsystem2/6(Out6) -> Subsystem3/6(Fb1)
  Subsystem4/1(Fc(t-tau)_actual) -> Scope16/1, Fc(t-tau)_actual/1
  Subsystem2/8(Out8) -> Subsystem3/8(Fb3)
  Subsystem1/2(Out2) -> Subsystem2/2(In2)
  Subsystem1/3(Out3) -> Subsystem2/3(In3)
  Subsystem2/7(Out7) -> Subsystem3/7(In7)
  Subsystem2/1(F_c_max) -> Subsystem3/1(In1)
  Subsystem2/3(Out3) -> Subsystem3/3(In3)
  Turn off for PID tune/1 -> Matrix Multiply5/2
  Subsystem1/1(Out1) -> Subsystem2/1(In1)
  Subsystem2/9(Out9) -> Subsystem3/9(In9)
  MATLAB Function5/3(F3) -> MATLAB Function4/3(F3)
  Matrix Multiply5/1 -> Subsystem/1(F_c_d)  "F_c_d"
  Subsystem3/2(Mc(t-tau)_actual) -> Mc(t-tau)_actual/1
  Subsystem3/1(Out1) -> Scope17/1, Subsystem4/2(In2)
  Subsystem/2(Ft_wanted) -> Subsystem1/2(In2)
  Subsystem2/4(Out4) -> Subsystem3/4(Ft3)
  MATLAB Function5/2(F2) -> MATLAB Function4/2(F2)
  Subsystem2/5(Out5) -> Subsystem3/5(Ft4)
  MATLAB Function5/1(F1) -> MATLAB Function4/1(F1)
  Fc(t-tau)/1 -> Turn off for PID tune/1
  Mcd/1 -> Gain6/1
  Subsystem/3(Fc_wanted) -> Subsystem1/3(In3)
  Subsystem4/2(Fc(t-tau)_actual1) -> Scope18/1
  Subsystem2/2(F_t_max) -> Subsystem3/2(In2)
  TVd/1 -> Subsystem4/1(TVd)
  Subsystem/1(Fb_wanted) -> Subsystem1/1(In1)

== system Trial_Merge_Unsuccessful/Subsystem11/Subsystem/Resettable Subsystem/Subsystem3 ==
  w^d : Inport
  a : Inport  Port=2
  T_dV : Inport  Port=3
  Add : Sum  Inputs=+-
  Add1 : Sum
  Demux21 : Demux  Outputs=3
  Demux22 : Demux  Outputs=3
  Gain : Gain  Gain=0
  Gain1 : Gain
  MATLAB Function10 : MATLAB Function  TreatAsAtomicUnit=on
  Matrix Multiply4 : Product  Multiplication=Matrix(*)
  Mux14 : Mux  Inputs=3
  To Workspace : ToWorkspace  VariableName=gyro  SaveFormat=Timeseries  SampleTime=-1
  w^d1 : Outport
  wires:
  Demux21/3 -> MATLAB Function10/3(zvel)
  Demux22/1 -> MATLAB Function10/4(accx)
  Demux22/2 -> MATLAB Function10/5(accy)
  Demux22/3 -> MATLAB Function10/6(accz)
  MATLAB Function10/1(wx) -> Mux14/1
  Demux21/1 -> MATLAB Function10/1(xvel)
  MATLAB Function10/2(wy) -> Mux14/2
  Demux21/2 -> MATLAB Function10/2(yvel)
  MATLAB Function10/3(wz) -> Mux14/3
  Matrix Multiply4/1 -> Demux22/1
  Mux14/1 -> Gain/1, Add/2  "w^d"
  T_dV/1 -> Matrix Multiply4/1
  a/1 -> Matrix Multiply4/2
  w^d/1 -> Gain1/1, Add/1, Demux21/1
  Add/1 -> To Workspace/1
  Gain/1 -> Add1/1
  Gain1/1 -> Add1/2
  Add1/1 -> w^d1/1

== system Trial_Merge_Unsuccessful/Subsystem11/Subsystem/Resettable Subsystem/Subsystem4 ==
  "theta, phi, psi" : Inport
  "sigma, tau, upsilon" : Inport  Port=2
  Demux6 : Demux  Outputs=3
  Demux7 : Demux  Outputs=3
  MATLAB Function2 : MATLAB Function  TreatAsAtomicUnit=on
  MATLAB Function3 : MATLAB Function  TreatAsAtomicUnit=on
  Matrix Multiply7 : Product  Multiplication=Matrix(*)
  Terminator{7..10} (4 alike) : Terminator
  Transpose4 : Math  Operator=transpose  SaturateOnIntegerOverflow=on
  Transpose5 : Math  Operator=transpose  SaturateOnIntegerOverflow=on
  Transpose6 : Math  Operator=transpose  SaturateOnIntegerOverflow=on
  T_dV : Outport
  T_Vd : Outport  Port=2
  wires:
  Matrix Multiply7/1 -> T_Vd/1, Transpose6/1  "T_Vd"
  Demux7/1 -> MATLAB Function3/1(theta_x)
  "theta, phi, psi"/1 -> Demux6/1
  Demux6/3 -> MATLAB Function2/3(theta_z)
  Demux7/3 -> MATLAB Function3/3(theta_z)
  "sigma, tau, upsilon"/1 -> Demux7/1
  Demux6/1 -> MATLAB Function2/1(theta_x)
  Transpose5/1 -> Terminator9/1, Matrix Multiply7/2  "T_Vt"
  MATLAB Function2/1(Transformation_Mat) -> Terminator7/1, Transpose4/1  "T_dt"
  Transpose4/1 -> Terminator8/1, Matrix Multiply7/1  "T_td"
  MATLAB Function3/1(Transformation_Mat) -> Terminator10/1, Transpose5/1  "T_tV"
  Demux6/2 -> MATLAB Function2/2(theta_y)
  Demux7/2 -> MATLAB Function3/2(theta_y)
  Transpose6/1 -> T_dV/1  "T_dV"

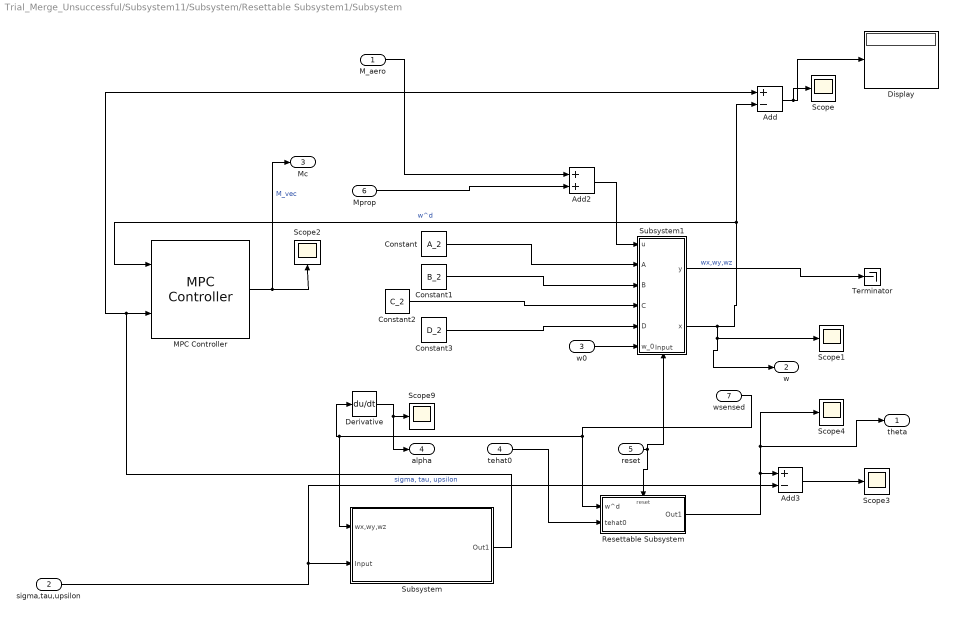
== system Trial_Merge_Unsuccessful/Subsystem11/Subsystem/Resettable Subsystem1/Subsystem ==
  M_aero : Inport
  sigma,tau,upsilon : Inport  Port=2
  w0 : Inport  Port=3
  tehat0 : Inport  Port=4
  reset : Inport  Port=5
  Mprop : Inport  Port=6
  wsensed : Inport  Port=7
  Add : Sum  Inputs=+-
  Add2 : Sum
  Add3 : Sum  Inputs=+-
  Constant : Constant  Value=A_2
  Constant1 : Constant  Value=B_2
  Constant2 : Constant  Value=C_2
  Constant3 : Constant  Value=D_2
  Derivative : Derivative
  Display : Display
  MPC Controller : mpclib/MPC Controller  SCDEnableBlockLinearizationSpecification=on  mpcobj=MPCDesignerSession.AppData.Controllers.MPC  is_multiple=0  enable_value=0  return_u0=off  updateMPCinCallerWorkspace=on  md_inport=off  mv_inport=off  uref_inport=off  return_cost=off  return_mvseq=off  return_qpstatus=off  return_xseq=off  return_state=off  return_ovseq=off  state_inport=off  umin_inport=off  umax_inport=off  ymin_inport=off  ymax_inport=off  cc_inport=off  ywt_inport=off  uwt_inport=off  duwt_inport=off  rhoeps_inport=off  pm_inport=off  MaximumP=10  HorizonChoice=FixedHorizon  n_ts=0.1  n_p=10  n_mv=3  n_md=0  n_ud=0  n_mo=3  n_uo=0  BlockDataType=double  SampleTimeInherited=off  switch_inport=off
  Resettable Subsystem : Subsystem  TreatAsAtomicUnit=on
  Scope{,1..4,9} (6 alike) : Scope
  Subsystem : Subsystem
  Subsystem1 : Subsystem
      settings: PortSchema="{\"entries\":[{\"content\":{\"sides\":[{\"content\":{\"connectorIds\":[\"In1\",\"In2\",\"In3\",\"In4\",\"In5\",\"In6\"]},\"type\":\"ConnectorPlacement.EquallySpacedRectSide\",\"uuid\":\"7d9460a7-3adf-4f89-91e7-b456f7078c86\"},{\"content\":{\"connectorIds\":[\"Out1\",\"Out2\"],\"side\":\"RIGHT\"},\"type\":\"ConnectorPlacement.EquallySpacedRectSide\",\"uuid\":\"f1bf29ac-ed67-4ce4-91e2-85f2b90efa08\"},{\"content\":{\"connectorIds\":[],\"side\":\"TOP\"},\"type\":\"ConnectorPlacement.EquallySpacedRectSide\",\"uuid\":\"d922c634-a6d8-424b-a167-3b858780e5fe\"},{\"content\":{\"connectorIds\":[\"In7\"],\"side\":\"BOTTOM\"},\"type\":\"ConnectorPlacement.EquallySpacedRectSide\",\"uuid\":\"f177f641-1570-409d-a38e-cef2b78f705f\"},{\"content\":{\"connectorIds\":[],\"side\":\"HIDDEN\"},\"type\":\"ConnectorPlacement.EquallySpacedRectSide\",\"uuid\":\"30cf80c6-7b26-40df-a778-919a6a544dd2\"}]},\"type\":\"ConnectorPlacement.EquallySpacedConnector\",\"uuid\":\"27252b95-3211-4624-87a6-4be9d32d6c6a\"}],\"packageUris\":[\"http://schema.mathworks.com/mf0/Connector/R2020b\"],\"version\":\"1.0\"}"
  Terminator : Terminator
  theta : Outport
  w : Outport  Port=2
  Mc : Outport  Port=3
  alpha : Outport  Port=4
  wires:
  Subsystem1/1(y) -> Terminator/1  "wx,wy,wz"
  Derivative/1 -> alpha/1, Scope9/1
  Resettable Subsystem/1(Out1) -> Scope4/1, theta/1, Add3/1
  Add/1 -> Display/1, Scope/1
  Add3/1 -> Scope3/1
  Add2/1 -> Subsystem1/1(u)
  sigma,tau,upsilon/1 -> Add3/2, Subsystem/2(Input)  "sigma, tau, upsilon"
  Subsystem/1(Out1) -> Add/1, MPC Controller/2
  M_aero/1 -> Add2/1
  Constant2/1 -> Subsystem1/4(C)
  Constant3/1 -> Subsystem1/5(D)
  Subsystem1/2(x) -> Add/2, MPC Controller/1, w/1, Scope1/1  "w^d"
  MPC Controller/1 -> Mc/1, Scope2/1  "M_vec"
  Constant/1 -> Subsystem1/2(A)
  Constant1/1 -> Subsystem1/3(B)
  w0/1 -> Subsystem1/6(w_0)
  tehat0/1 -> Resettable Subsystem/2(tehat0)
  reset/1 -> Subsystem1/7(Input), Resettable Subsystem/Reset
  Mprop/1 -> Add2/2
  wsensed/1 -> Resettable Subsystem/1(w^d), Subsystem/1(wx,wy,wz), Derivative/1

== system Trial_Merge_Unsuccessful/Subsystem11/Subsystem/Resettable Subsystem1/Subsystem1 ==
  Mcd : Inport
  Fc(t-tau) : Inport  Port=2
  Tvd : Inport  Port=3
  TVd : Inport  Port=4
  Gain6 : Gain
  MATLAB Function4 : MATLAB Function  Commented=on  TreatAsAtomicUnit=on
  MATLAB Function5 : MATLAB Function  Commented=on  TreatAsAtomicUnit=on
  Matrix Multiply5 : Product  Multiplication=Matrix(*)
  Scope16 : Scope
  Scope17 : Scope
  Scope18 : Scope
  Subsystem : Subsystem
  Subsystem1 : Subsystem
  Subsystem2 : Subsystem
  Subsystem3 : Subsystem
  Subsystem4 : Subsystem
  Turn off for PID tune : Gain
  Mc(t-tau)_actual : Outport
  Fc(t-tau)_actual : Outport  Port=2
  wires:
  Gain6/1 -> Subsystem/2(M_c_d)  "M_c_d"
  Tvd/1 -> Matrix Multiply5/1
  Subsystem2/6(Out6) -> Subsystem3/6(Fb1)
  Subsystem4/1(Fc(t-tau)_actual) -> Scope16/1, Fc(t-tau)_actual/1
  Subsystem2/8(Out8) -> Subsystem3/8(Fb3)
  Subsystem1/2(Out2) -> Subsystem2/2(In2)
  Subsystem1/3(Out3) -> Subsystem2/3(In3)
  Subsystem2/7(Out7) -> Subsystem3/7(In7)
  Subsystem2/1(F_c_max) -> Subsystem3/1(In1)
  Subsystem2/3(Out3) -> Subsystem3/3(In3)
  Turn off for PID tune/1 -> Matrix Multiply5/2
  Subsystem1/1(Out1) -> Subsystem2/1(In1)
  Subsystem2/9(Out9) -> Subsystem3/9(In9)
  MATLAB Function5/3(F3) -> MATLAB Function4/3(F3)
  Matrix Multiply5/1 -> Subsystem/1(F_c_d)  "F_c_d"
  Subsystem3/2(Mc(t-tau)_actual) -> Mc(t-tau)_actual/1
  Subsystem3/1(Out1) -> Scope17/1, Subsystem4/2(In2)
  Subsystem/2(Ft_wanted) -> Subsystem1/2(In2)
  Subsystem2/4(Out4) -> Subsystem3/4(Ft3)
  MATLAB Function5/2(F2) -> MATLAB Function4/2(F2)
  Subsystem2/5(Out5) -> Subsystem3/5(Ft4)
  MATLAB Function5/1(F1) -> MATLAB Function4/1(F1)
  Fc(t-tau)/1 -> Turn off for PID tune/1
  Mcd/1 -> Gain6/1
  Subsystem/3(Fc_wanted) -> Subsystem1/3(In3)
  Subsystem4/2(Fc(t-tau)_actual1) -> Scope18/1
  Subsystem2/2(F_t_max) -> Subsystem3/2(In2)
  TVd/1 -> Subsystem4/1(TVd)
  Subsystem/1(Fb_wanted) -> Subsystem1/1(In1)

== system Trial_Merge_Unsuccessful/Subsystem11/Subsystem/Resettable Subsystem1/Subsystem3 ==
  w^d : Inport
  a : Inport  Port=2
  T_dV : Inport  Port=3
  Add : Sum  Inputs=+-
  Add1 : Sum
  Demux21 : Demux  Outputs=3
  Demux22 : Demux  Outputs=3
  Gain : Gain  Gain=0
  Gain1 : Gain
  MATLAB Function10 : MATLAB Function  TreatAsAtomicUnit=on
  Matrix Multiply4 : Product  Multiplication=Matrix(*)
  Mux14 : Mux  Inputs=3
  To Workspace : ToWorkspace  VariableName=gyro  SaveFormat=Timeseries  SampleTime=-1
  w^d1 : Outport
  wires:
  Demux21/3 -> MATLAB Function10/3(zvel)
  Demux22/1 -> MATLAB Function10/4(accx)
  Demux22/2 -> MATLAB Function10/5(accy)
  Demux22/3 -> MATLAB Function10/6(accz)
  MATLAB Function10/1(wx) -> Mux14/1
  Demux21/1 -> MATLAB Function10/1(xvel)
  MATLAB Function10/2(wy) -> Mux14/2
  Demux21/2 -> MATLAB Function10/2(yvel)
  MATLAB Function10/3(wz) -> Mux14/3
  Matrix Multiply4/1 -> Demux22/1
  Mux14/1 -> Gain/1, Add/2  "w^d"
  T_dV/1 -> Matrix Multiply4/1
  a/1 -> Matrix Multiply4/2
  w^d/1 -> Gain1/1, Add/1, Demux21/1
  Add/1 -> To Workspace/1
  Gain/1 -> Add1/1
  Gain1/1 -> Add1/2
  Add1/1 -> w^d1/1

== system Trial_Merge_Unsuccessful/Subsystem11/Subsystem/Resettable Subsystem1/Subsystem4 ==
  "theta, phi, psi" : Inport
  "sigma, tau, upsilon" : Inport  Port=2
  Demux6 : Demux  Outputs=3
  Demux7 : Demux  Outputs=3
  MATLAB Function2 : MATLAB Function  TreatAsAtomicUnit=on
  MATLAB Function3 : MATLAB Function  TreatAsAtomicUnit=on
  Matrix Multiply7 : Product  Multiplication=Matrix(*)
  Terminator{7..10} (4 alike) : Terminator
  Transpose4 : Math  Operator=transpose  SaturateOnIntegerOverflow=on
  Transpose5 : Math  Operator=transpose  SaturateOnIntegerOverflow=on
  Transpose6 : Math  Operator=transpose  SaturateOnIntegerOverflow=on
  T_dV : Outport
  T_Vd : Outport  Port=2
  wires:
  Matrix Multiply7/1 -> T_Vd/1, Transpose6/1  "T_Vd"
  Demux7/1 -> MATLAB Function3/1(theta_x)
  "theta, phi, psi"/1 -> Demux6/1
  Demux6/3 -> MATLAB Function2/3(theta_z)
  Demux7/3 -> MATLAB Function3/3(theta_z)
  "sigma, tau, upsilon"/1 -> Demux7/1
  Demux6/1 -> MATLAB Function2/1(theta_x)
  Transpose5/1 -> Terminator9/1, Matrix Multiply7/2  "T_Vt"
  MATLAB Function2/1(Transformation_Mat) -> Terminator7/1, Transpose4/1  "T_dt"
  Transpose4/1 -> Terminator8/1, Matrix Multiply7/1  "T_td"
  MATLAB Function3/1(Transformation_Mat) -> Terminator10/1, Transpose5/1  "T_tV"
  Demux6/2 -> MATLAB Function2/2(theta_y)
  Demux7/2 -> MATLAB Function3/2(theta_y)
  Transpose6/1 -> T_dV/1  "T_dV"

== system Trial_Merge_Unsuccessful/Subsystem11/Subsystem/Resettable Subsystem/Subsystem/Subsystem ==
  F_c_d : Inport
  M_c_d : Inport  Port=2
  Demux8 : Demux  Outputs=3
  Demux9 : Demux  Outputs=3
  MATLAB Function : MATLAB Function  TreatAsAtomicUnit=on
  MATLAB Function6 : MATLAB Function  TreatAsAtomicUnit=on
  Mux23 : Mux
  Mux24 : Mux
  Mux9 : Mux  Inputs=3
  Terminator12 : Terminator
  To Workspace6 : ToWorkspace  VariableName=Fc_wanted  SaveFormat=Timeseries  SampleTime=-1
  To Workspace7 : ToWorkspace  VariableName=Ft_wanted  SaveFormat=Timeseries  SampleTime=-1
  To Workspace8 : ToWorkspace  VariableName=Fb_wanted  SaveFormat=Timeseries  SampleTime=-1
  Fb_wanted : Outport
  Ft_wanted : Outport  Port=2
  Fc_wanted : Outport  Port=3
  wires:
  Demux9/3 -> MATLAB Function6/3(M_z)
  Demux8/2 -> MATLAB Function6/1(F_y)
  Mux9/1 -> Fc_wanted/1, To Workspace6/1  "Fc_wanted"
  MATLAB Function/2(Ft2) -> Mux23/2  "Fb_wanted"
  Demux9/1 -> MATLAB Function6/2(M_x)
  MATLAB Function/3(Ft3) -> Mux23/3
  Demux9/2 -> MATLAB Function/1(My)
  MATLAB Function/8(Fb4) -> Mux24/4
  MATLAB Function6/1(F_c1) -> Mux9/1
  MATLAB Function/1(Ft1) -> Mux23/1  "Ft_wanted"
  Demux8/1 -> Terminator12/1
  Mux23/1 -> Ft_wanted/1, To Workspace7/1  "Ft_wanted"
  Mux24/1 -> Fb_wanted/1, To Workspace8/1  "Fb_wanted"
  MATLAB Function6/3(F_c3) -> Mux9/3
  MATLAB Function/5(Fb1) -> Mux24/1
  MATLAB Function/6(Fb2) -> Mux24/2
  MATLAB Function/7(Fb3) -> Mux24/3
  MATLAB Function/4(Ft4) -> Mux23/4
  Demux8/3 -> MATLAB Function/2(Fz)
  MATLAB Function6/2(F_c2) -> Mux9/2
  F_c_d/1 -> Demux8/1
  M_c_d/1 -> Demux9/1

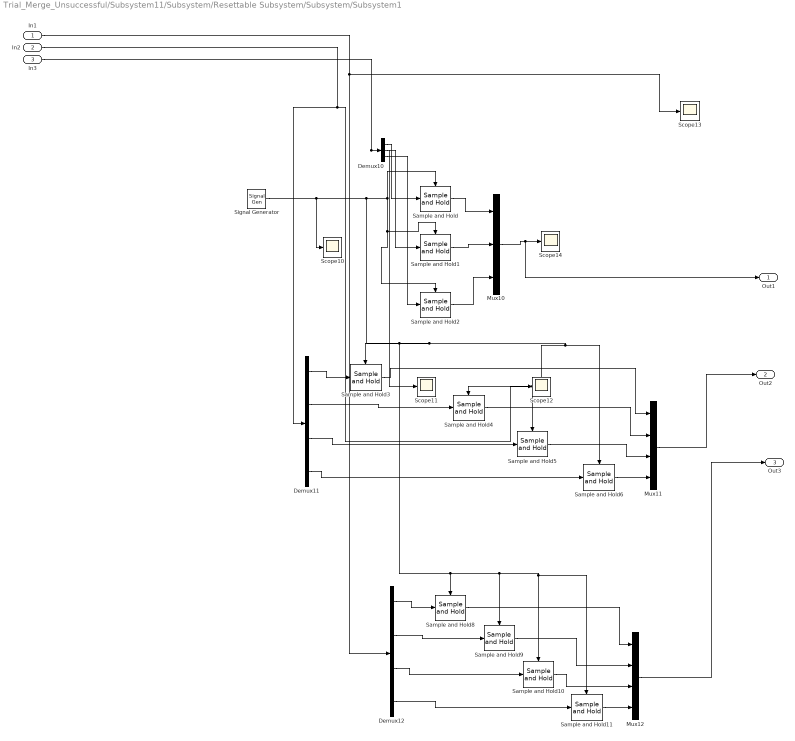
== system Trial_Merge_Unsuccessful/Subsystem11/Subsystem/Resettable Subsystem/Subsystem/Subsystem1 ==
  In1 : Inport
  In2 : Inport  Port=2
  In3 : Inport  Port=3
  Demux10 : Demux  Outputs=3
  Demux11 : Demux
  Demux12 : Demux
  Mux10 : Mux  Inputs=3
  Mux11 : Mux
  Mux12 : Mux
  Sample and Hold{,1..6,8..11} (11 alike) : dspsigops/Sample and Hold  trig=Rising edge  initCond=0  latchinput=off
  Scope{10..14} (5 alike) : Scope
  Signal Generator : SignalGenerator  WaveForm=square  Frequency=fprop  Units=rad/sec
  Out1 : Outport
  Out2 : Outport  Port=2
  Out3 : Outport  Port=3
  wires:
  Demux12/1 -> Sample and Hold8/1
  Demux11/1 -> Sample and Hold3/1
  Signal Generator/1 -> Scope10/1, Sample and Hold11/Trigger, Sample and Hold10/Trigger, Sample and Hold9/Trigger, Sample and Hold8/Trigger, Sample and Hold4/Trigger, Sample and Hold5/Trigger, Sample and Hold6/Trigger, Sample and Hold3/Trigger, Sample and Hold/Trigger, Sample and Hold2/Trigger, Sample and Hold1/Trigger
  In2/1 -> Scope12/1, Demux11/1
  In3/1 -> Scope11/1, Demux10/1
  Demux10/3 -> Sample and Hold2/1
  Sample and Hold10/1 -> Mux12/3
  Sample and Hold/1 -> Mux10/1
  Demux12/4 -> Sample and Hold11/1
  Sample and Hold6/1 -> Mux11/4
  Demux10/1 -> Sample and Hold/1
  Mux10/1 -> Out1/1, Scope14/1
  Demux12/3 -> Sample and Hold10/1
  Sample and Hold8/1 -> Mux12/1
  Sample and Hold3/1 -> Mux11/1
  Sample and Hold5/1 -> Mux11/3
  Sample and Hold1/1 -> Mux10/2
  Sample and Hold11/1 -> Mux12/4
  In1/1 -> Scope13/1, Demux12/1
  Demux10/2 -> Sample and Hold1/1
  Demux11/2 -> Sample and Hold4/1
  Sample and Hold2/1 -> Mux10/3
  Sample and Hold4/1 -> Mux11/2
  Sample and Hold9/1 -> Mux12/2
  Demux11/3 -> Sample and Hold5/1
  Mux12/1 -> Out3/1
  Demux12/2 -> Sample and Hold9/1
  Demux11/4 -> Sample and Hold6/1
  Mux11/1 -> Out2/1

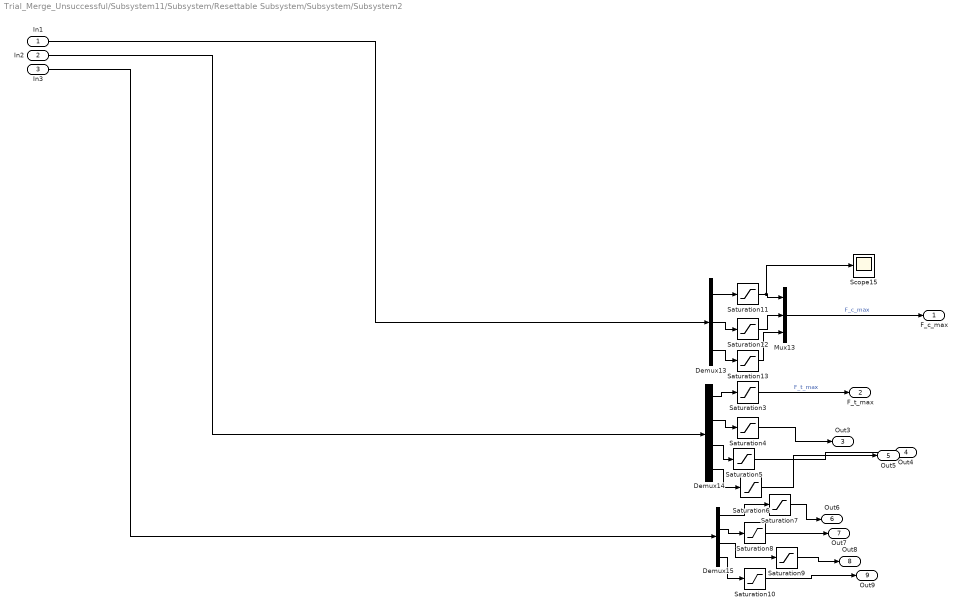
== system Trial_Merge_Unsuccessful/Subsystem11/Subsystem/Resettable Subsystem/Subsystem/Subsystem2 ==
  In1 : Inport
  In2 : Inport  Port=2
  In3 : Inport  Port=3
  Demux13 : Demux  Outputs=3
  Demux14 : Demux
  Demux15 : Demux
  Mux13 : Mux  Inputs=3
  Saturation10 : Saturate  UpperLimit=Fb4_u  LowerLimit=Fb4_l
  Saturation11 : Saturate  UpperLimit=Fc1_u  LowerLimit=Fc1_l
  Saturation12 : Saturate  UpperLimit=Fc2_u  LowerLimit=Fc2_l
  Saturation13 : Saturate  UpperLimit=Fc3_u  LowerLimit=Fc3_l
  Saturation3 : Saturate  UpperLimit=Ft1_u  LowerLimit=Ft1_l
  Saturation4 : Saturate  UpperLimit=Ft2_u  LowerLimit=Ft2_l
  Saturation5 : Saturate  UpperLimit=Ft3_u  LowerLimit=Ft3_l
  Saturation6 : Saturate  UpperLimit=Ft4_u  LowerLimit=Ft4_l
  Saturation7 : Saturate  UpperLimit=Fb1_u  LowerLimit=Fb1_l
  Saturation8 : Saturate  UpperLimit=Fb2_u  LowerLimit=Fb2_l
  Saturation9 : Saturate  UpperLimit=Fb3_u  LowerLimit=Fb3_l
  Scope15 : Scope
  F_c_max : Outport
  F_t_max : Outport  Port=2
  Out3 : Outport  Port=3
  Out4 : Outport  Port=4
  Out5 : Outport  Port=5
  Out6 : Outport  Port=6
  Out7 : Outport  Port=7
  Out8 : Outport  Port=8
  Out9 : Outport  Port=9
  wires:
  Saturation11/1 -> Scope15/1, Mux13/1
  Demux13/2 -> Saturation12/1
  Saturation10/1 -> Out9/1
  Demux13/3 -> Saturation13/1
  Demux14/1 -> Saturation3/1
  Demux14/4 -> Saturation6/1
  In3/1 -> Demux15/1
  Demux14/3 -> Saturation5/1
  Demux13/1 -> Saturation11/1
  Saturation13/1 -> Mux13/3
  In1/1 -> Demux13/1
  Demux15/1 -> Saturation7/1
  Demux15/2 -> Saturation8/1
  Demux15/3 -> Saturation9/1
  Saturation12/1 -> Mux13/2
  Demux15/4 -> Saturation10/1
  Demux14/2 -> Saturation4/1
  Saturation9/1 -> Out8/1
  Saturation5/1 -> Out4/1
  In2/1 -> Demux14/1
  Saturation4/1 -> Out3/1
  Saturation7/1 -> Out6/1
  Mux13/1 -> F_c_max/1  "F_c_max"
  Saturation6/1 -> Out5/1
  Saturation3/1 -> F_t_max/1  "F_t_max"
  Saturation8/1 -> Out7/1

== system Trial_Merge_Unsuccessful/Subsystem11/Subsystem/Resettable Subsystem/Subsystem/Subsystem3 ==
  In1 : Inport
  In2 : Inport  Port=2
  In3 : Inport  Port=3
  Ft3 : Inport  Port=4
  Ft4 : Inport  Port=5
  Fb1 : Inport  Port=6
  In7 : Inport  Port=7
  Fb3 : Inport  Port=8
  In9 : Inport  Port=9
  Constant23 : Constant  Value=0
  Demux16 : Demux  Outputs=3
  MATLAB Function7 : MATLAB Function  TreatAsAtomicUnit=on
  MATLAB Function8 : MATLAB Function  TreatAsAtomicUnit=on
  MATLAB Function9 : MATLAB Function  TreatAsAtomicUnit=on
  Mux : Mux
  Mux1 : Mux
  Mux16 : Mux  Inputs=3
  Mux17 : Mux  Inputs=3
  To Workspace : ToWorkspace  VariableName=Fc  SaveFormat=Timeseries  SampleTime=-1
  To Workspace1 : ToWorkspace  VariableName=Ft  SaveFormat=Timeseries  SampleTime=-1
  To Workspace2 : ToWorkspace  VariableName=Fb  SaveFormat=Timeseries  SampleTime=-1
  Out1 : Outport
  Mc(t-tau)_actual : Outport  Port=2
  wires:
  Demux16/2 -> MATLAB Function8/2(F_c2)
  In9/1 -> Mux1/4, MATLAB Function9/8(Fb4)
  In3/1 -> Mux/2, MATLAB Function9/2(Ft2)
  MATLAB Function7/1(F_z) -> Mux16/3  "Fz_actual"
  In1/1 -> Demux16/1, To Workspace/1
  Fb3/1 -> Mux1/3, MATLAB Function9/7(Fb3)
  MATLAB Function9/1(F1) -> MATLAB Function7/1(F1)
  Ft3/1 -> Mux/3, MATLAB Function9/3(Ft3)
  MATLAB Function8/1(F_y) -> Mux16/2  "Fy_actual"
  Fb1/1 -> Mux1/1, MATLAB Function9/5(Fb1)
  MATLAB Function8/3(M_z) -> Mux17/3  "M_z_acc"
  MATLAB Function7/2(M_y) -> Mux17/2  "M_y_acc"
  Mux17/1 -> Mc(t-tau)_actual/1  "Mc(t-tau)_actual"
  Ft4/1 -> Mux/4, MATLAB Function9/4(Ft4)
  MATLAB Function8/2(M_x) -> Mux17/1  "M_x_acc"
  In7/1 -> Mux1/2, MATLAB Function9/6(Fb2)
  MATLAB Function9/3(F3) -> MATLAB Function7/3(F3)
  Demux16/1 -> MATLAB Function8/1(F_c1)
  Constant23/1 -> Mux16/1  "Fx_actual"
  In2/1 -> Mux/1, MATLAB Function9/1(Ft1)
  MATLAB Function9/2(F2) -> MATLAB Function7/2(F2)
  Mux1/1 -> To Workspace2/1
  Demux16/3 -> MATLAB Function8/3(F_c3)
  Mux/1 -> To Workspace1/1
  Mux16/1 -> Out1/1

== system Trial_Merge_Unsuccessful/Subsystem11/Subsystem/Resettable Subsystem/Subsystem/Subsystem4 ==
  TVd : Inport
  In2 : Inport  Port=2
  Constant24 : Constant  Value=[0;1;1]
  Matrix Multiply3 : Product  Multiplication=Matrix(*)
  Product5 : Product
  Fc(t-tau)_actual : Outport
  Fc(t-tau)_actual1 : Outport  Port=2
  wires:
  Matrix Multiply3/1 -> Fc(t-tau)_actual1/1, Product5/2  "Fc(t-tau)_actual"
  Constant24/1 -> Product5/1
  TVd/1 -> Matrix Multiply3/1
  Product5/1 -> Fc(t-tau)_actual/1  "Fc(t-tau)_actual"
  In2/1 -> Matrix Multiply3/2

== system Trial_Merge_Unsuccessful/Subsystem11/Subsystem/Resettable Subsystem1/Subsystem/Resettable Subsystem ==
  w^d : Inport
  tehat0 : Inport  Port=2
  Reset : ResetPort  DisableCoverage=on
  Integrator : Integrator  InitialConditionSource=external  InitialCondition=theta0
  Scope : Scope
  Out1 : Outport
  wires:
  tehat0/1 -> Integrator/2
  w^d/1 -> Integrator/1
  Integrator/1 -> Scope/1, Out1/1
